simulink model "test_rx_err_cnt"  (Simulink 6.2)
settings: Solver=ode45  StartTime=0.0  StopTime=1000  RelTol=1e-3
libraries: xbsIndex_r3 x58, xps_library x6, casper_library x2
settings Model: LastModifiedBy=dsp
settings DebuggingCC: SolverPrmCheckMsg=warning

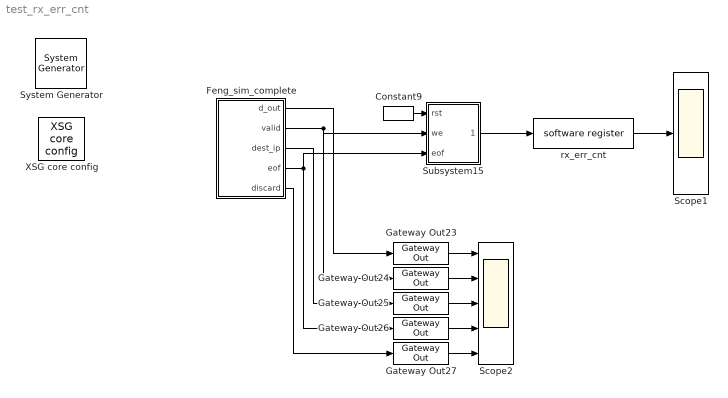
== system test_rx_err_cnt ==
  " System Generator" : xbsIndex_r3/ System Generator  Tag=genX  xilinxfamily=Virtex2P  part=xc2vp70  speed=-7  package=ff1704  synthesis_tool=XST  directory=./b_2x_8a_r308d/sysgen  testbench=off  simulink_period=1  sysclk_period=4.878  incr_netlist=off  trim_vbits=Everywhere in SubSystem  dbl_ovrd=According to Block Masks  core_generation=According to Block Masks  run_coregen=off  deprecated_control=off  eval_field=0
      settings: AttributesFormatString=System\nGenerator
  Constant9 : xbsIndex_r3/Constant  const=0  equ=P=C  arith_type=Boolean  n_bits=1  bin_pt=0  opselect=C  inp2=PCIN>>17  opr=+  inp1=P  carry=CIN  iostate=0  explicit_period=on  period=1  dbl_ovrd=off
  Feng_sim_complete : Subsystem
  Gateway Out{23..27} (5 alike) : xbsIndex_r3/Gateway Out  output_type=Double  nbits=8  bin_pt=6  arith_type=Boolean  quantization=Truncate  overflow=Wrap  hdl_port=on  timing_constraint=None  locs_specified=off  LOCs={}  needs_fixed_name=off  show_param=off
      settings: xl_area=[0, 0, 0, 0, 0, 0, 0]
  Scope1 : Scope
      settings: TimeRange=10000  YMin=0  YMax=5000
  Scope2 : Scope  NumInputPorts=5
      settings: TimeRange=10000  YMin=0~0~0~0~-1  YMax=5000~1~3~1~1
  Subsystem15 : Subsystem  mask{payload_len=51}
      mask init:
      | fmtstr = sprintf('Payload Length: %d', payload_len);
      | set_param(gcb, 'AttributesFormatString', fmtstr);
      settings: AttributesFormatString=Payload Length: 51
  XSG core config : xps_library/XSG core config  Tag=xps:xsg  hw_sys=BEE2_usr  ibob_linux=off  clk_src=sys_clk2x  gpio_clk_io_group=iBOB:sma  gpio_clk_bit_index=0  clk_rate=205  sample_period=1  synthesis_tool=XST  mpc_type=powerpc405
  rx_err_cnt : xps_library/software register  Tag=xps:sw_reg  io_dir=To Processor  arith_type=Unsigned  bitwidth=32  bin_pt=0  sample_period=1  gw_name=test_rx_err_cnt_rx_err_cnt_user_data_in
  wires:
  Subsystem15/1(err_cnt) -> rx_err_cnt/1
  Constant9/1 -> Subsystem15/1(rst)
  Gateway Out23/1 -> Scope2/1
  Gateway Out24/1 -> Scope2/2
  Gateway Out25/1 -> Scope2/3
  Gateway Out26/1 -> Scope2/4
  Gateway Out27/1 -> Scope2/5
  Feng_sim_complete/1(d_out) -> Gateway Out23/1
  Feng_sim_complete/2(valid) -> Gateway Out24/1, Subsystem15/2(we)
  Feng_sim_complete/3(dest_ip) -> Gateway Out25/1
  Feng_sim_complete/4(eof) -> Gateway Out26/1, Subsystem15/3(eof)
  Feng_sim_complete/5(discard) -> Gateway Out27/1
  rx_err_cnt/1 -> Scope1/1

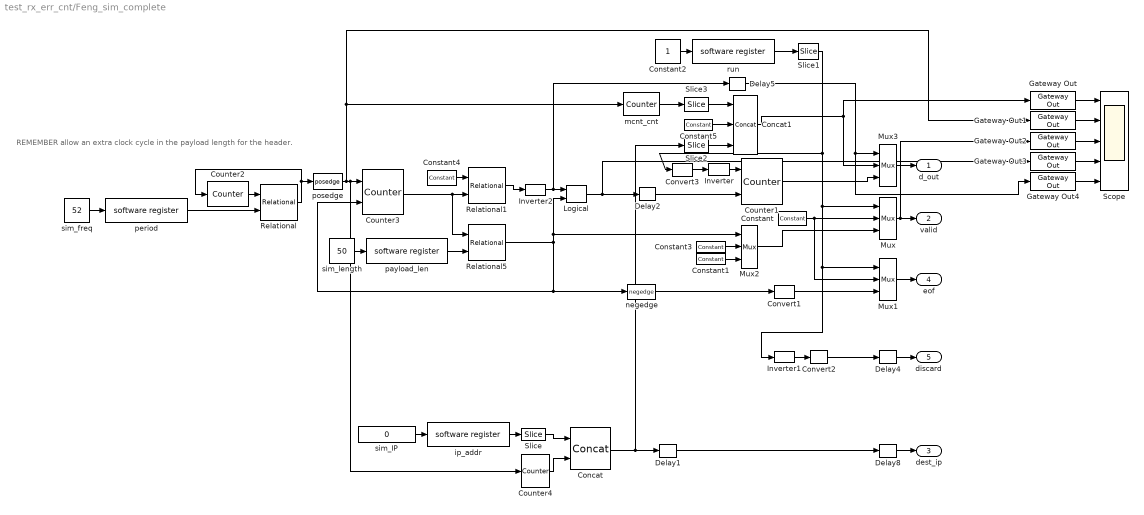
== system test_rx_err_cnt/Feng_sim_complete ==
  note: REMEMBER
      | allow an extra clock cycle in the
      | payload length for the header.
  Concat : xbsIndex_r3/Concat  num_inputs=2  explicit_period=off  period=1  dbl_ovrd=off
  Concat1 : xbsIndex_r3/Concat  num_inputs=3  explicit_period=off  period=1  dbl_ovrd=off
  Constant : xbsIndex_r3/Constant  const=0  equ=P=C  arith_type=Boolean  n_bits=1  bin_pt=0  opselect=C  inp2=PCIN>>17  opr=+  inp1=P  carry=CIN  iostate=0  explicit_period=on  period=1  dbl_ovrd=off
  Constant1 : xbsIndex_r3/Constant  const=1  equ=P=C  arith_type=Boolean  n_bits=1  bin_pt=0  opselect=C  inp2=PCIN>>17  opr=+  inp1=P  carry=CIN  iostate=0  explicit_period=off  period=1  dbl_ovrd=off
  Constant2 : Constant
  Constant3 : xbsIndex_r3/Constant  const=0  equ=P=C  arith_type=Boolean  n_bits=1  bin_pt=0  opselect=C  inp2=PCIN>>17  opr=+  inp1=P  carry=CIN  iostate=0  explicit_period=off  period=1  dbl_ovrd=off
  Constant4 : xbsIndex_r3/Constant  const=0  equ=P=C  arith_type=Unsigned  n_bits=32  bin_pt=0  opselect=C  inp2=PCIN>>17  opr=+  inp1=P  carry=CIN  iostate=0  explicit_period=on  period=1  dbl_ovrd=off
  Constant5 : xbsIndex_r3/Constant  const=0  equ=P=C  arith_type=Unsigned  n_bits=16-2  bin_pt=0  opselect=C  inp2=PCIN>>17  opr=+  inp1=P  carry=CIN  iostate=0  explicit_period=on  period=1  dbl_ovrd=off
  Convert1 : xbsIndex_r3/Convert  arith_type=Boolean  n_bits=8  bin_pt=6  quantization=Truncate  overflow=Wrap  latency=0  explicit_period=on  period=1  dbl_ovrd=off  show_param=off  inserted_by_tool=off  pipeline=off
      settings: xl_area=[0, 0, 0, 0, 0, 0, 0]
  Convert2 : xbsIndex_r3/Convert  arith_type=Boolean  n_bits=8  bin_pt=6  quantization=Truncate  overflow=Wrap  latency=0  explicit_period=on  period=1  dbl_ovrd=off  show_param=off  inserted_by_tool=off  pipeline=off
      settings: xl_area=[0, 0, 0, 0, 0, 0, 0]
  Convert3 : xbsIndex_r3/Convert  arith_type=Boolean  n_bits=8  bin_pt=6  quantization=Truncate  overflow=Wrap  latency=0  explicit_period=on  period=1  dbl_ovrd=off  show_param=off  inserted_by_tool=off  pipeline=off
      settings: xl_area=[0, 0, 0, 0, 0, 0, 0]
  Counter1 : xbsIndex_r3/Counter  cnt_type=Free Running  n_bits=64  bin_pt=0  arith_type=Unsigned  start_count=0  cnt_to=Inf  cnt_by_val=1  operation=Up  explicit_period=off  period=1  load_pin=off  rst=on  en=on  dbl_ovrd=off  show_param=off  use_rpm=off  gen_core=off
      settings: xl_area=[0, 0, 0, 0, 0, 0, 0]
  Counter2 : xbsIndex_r3/Counter  cnt_type=Free Running  n_bits=32  bin_pt=0  arith_type=Unsigned  start_count=1  cnt_to=Inf  cnt_by_val=1  operation=Up  explicit_period=on  period=1  load_pin=off  rst=on  en=off  dbl_ovrd=off  show_param=off  use_rpm=on  gen_core=off
      settings: xl_area=[0, 0, 0, 0, 0, 0, 0]
  Counter3 : xbsIndex_r3/Counter  cnt_type=Free Running  n_bits=32  bin_pt=0  arith_type=Unsigned  start_count=0  cnt_to=1023  cnt_by_val=1  operation=Up  explicit_period=on  period=1  load_pin=off  rst=on  en=on  dbl_ovrd=off  show_param=off  use_rpm=on  gen_core=off
      settings: xl_area=[0, 0, 0, 0, 0, 0, 0]
  Counter4 : xbsIndex_r3/Counter  cnt_type=Free Running  n_bits=2  bin_pt=0  arith_type=Unsigned  start_count=0  cnt_to=1023  cnt_by_val=1  operation=Up  explicit_period=on  period=1  load_pin=off  rst=off  en=on  dbl_ovrd=off  show_param=off  use_rpm=on  gen_core=off
      settings: xl_area=[0, 0, 0, 0, 0, 0, 0]
  Delay{1..2,4..5,8} (5 alike) : xbsIndex_r3/Delay  latency=1  reg_retiming=on  explicit_period=off  period=1  en=off  accept_only_valid=off  init_zero=on  dbl_ovrd=off  show_param=off
      settings: xl_area=[0, 0, 0, 0, 0, 0, 0]
  Gateway Out{,1..4} (5 alike) : xbsIndex_r3/Gateway Out  output_type=Double  nbits=8  bin_pt=6  arith_type=Boolean  quantization=Truncate  overflow=Wrap  hdl_port=on  timing_constraint=None  locs_specified=off  LOCs={}  needs_fixed_name=off  show_param=off
      settings: xl_area=[0, 0, 0, 0, 0, 0, 0]
  Inverter : xbsIndex_r3/Inverter  latency=0  explicit_period=off  period=1  en=off  dbl_ovrd=off  show_param=off
      settings: xl_area=[0, 0, 0, 0, 0, 0, 0]
  Inverter1 : xbsIndex_r3/Inverter  latency=0  explicit_period=off  period=1  en=off  dbl_ovrd=off  show_param=off
      settings: xl_area=[0, 0, 0, 0, 0, 0, 0]
  Inverter2 : xbsIndex_r3/Inverter  latency=0  explicit_period=off  period=1  en=off  dbl_ovrd=off  show_param=off
      settings: xl_area=[0, 0, 0, 0, 0, 0, 0]
  Logical : xbsIndex_r3/Logical  logical_function=AND  inputs=2  precision=Full  arith_type=Unsigned  n_bits=8  bin_pt=2  align_bp=on  latency=0  explicit_period=off  period=1  en=off  dbl_ovrd=off  show_param=off
      settings: xl_area=[0, 0, 0, 0, 0, 0, 0]
  Mux{,1..3} (4 alike) : xbsIndex_r3/Mux  inputs=2  precision=Full  arith_type="Signed  (2's comp)"  n_bits=8  bin_pt=2  quantization=Truncate  overflow=Wrap  latency=1  explicit_period=off  period=1  en=off  dbl_ovrd=off  show_param=off  mux_type=off  use_rpm=off  gen_core=off
      settings: xl_area=[0, 0, 0, 0, 0, 0, 0]
  Relational : xbsIndex_r3/Relational  mode=a>=b  latency=0  explicit_period=on  period=1  en=off  dbl_ovrd=off  show_param=off
      settings: xl_area=[0, 0, 0, 0, 0, 0, 0]
  Relational1 : xbsIndex_r3/Relational  mode=a=b  latency=0  explicit_period=off  period=1  en=off  dbl_ovrd=off  show_param=off
      settings: xl_area=[0, 0, 0, 0, 0, 0, 0]
  Relational5 : xbsIndex_r3/Relational  mode=a<=b  latency=0  explicit_period=off  period=1  en=off  dbl_ovrd=off  show_param=off
      settings: xl_area=[0, 0, 0, 0, 0, 0, 0]
  Scope : Scope  NumInputPorts=5
      settings: TimeRange=4000  YMin=130000~0~0~0~0  YMax=200000~1~1~1~1  SaveName=ScopeData11
  Slice : xbsIndex_r3/Slice  mode=Upper Bit Location + Width  nbits=30  bit1=0  base1=MSB of Input  bit0=0  base0=LSB of Input  boolean_output=off  explicit_period=off  period=1  dbl_ovrd=off
  Slice1 : xbsIndex_r3/Slice  mode=Lower Bit Location + Width  nbits=1  bit1=1  base1=MSB of Input  bit0=0  base0=LSB of Input  boolean_output=off  explicit_period=off  period=1  dbl_ovrd=off
  Slice2 : xbsIndex_r3/Slice  mode=Lower Bit Location + Width  nbits=2  bit1=1  base1=MSB of Input  bit0=0  base0=LSB of Input  boolean_output=off  explicit_period=off  period=1  dbl_ovrd=off
  Slice3 : xbsIndex_r3/Slice  mode=Lower Bit Location + Width  nbits=48  bit1=1  base1=MSB of Input  bit0=3  base0=LSB of Input  boolean_output=off  explicit_period=off  period=1  dbl_ovrd=off
  ip_addr : xps_library/software register  Tag=xps:sw_reg  io_dir=From Processor  arith_type=Unsigned  bitwidth=32  bin_pt=0  sample_period=1  gw_name=test_rx_err_cnt_Feng_sim_complete_ip_addr_user_data_out
  mcnt_cnt : xbsIndex_r3/Counter  cnt_type=Free Running  n_bits=64  bin_pt=0  arith_type=Unsigned  start_count=0  cnt_to=Inf  cnt_by_val=1  operation=Up  explicit_period=off  period=1  load_pin=off  rst=off  en=on  dbl_ovrd=off  show_param=off  use_rpm=off  gen_core=off
      settings: xl_area=[0, 0, 0, 0, 0, 0, 0]
  negedge : casper_library/Misc/negedge  Tag=Rising Edge Detector
  payload_len : xps_library/software register  Tag=xps:sw_reg  io_dir=From Processor  arith_type=Unsigned  bitwidth=32  bin_pt=0  sample_period=1  gw_name=test_rx_err_cnt_Feng_sim_complete_payload_len_user_data_out
  period : xps_library/software register  Tag=xps:sw_reg  io_dir=From Processor  arith_type=Unsigned  bitwidth=32  bin_pt=0  sample_period=1  gw_name=test_rx_err_cnt_Feng_sim_complete_period_user_data_out
  posedge : casper_library/Misc/pulse_ext/posedge  Tag=Rising Edge Detector
  run : xps_library/software register  Tag=xps:sw_reg  io_dir=From Processor  arith_type=Unsigned  bitwidth=32  bin_pt=0  sample_period=1  gw_name=test_rx_err_cnt_Feng_sim_complete_run_user_data_out
  sim_IP : Constant  Value=0
  sim_freq : Constant  Value=52
  sim_length : Constant  Value=50
  d_out : Outport
  valid : Outport  Port=2
  dest_ip : Outport  Port=3
  eof : Outport  Port=4
  discard : Outport  Port=5
  wires:
  Delay1/1 -> Delay8/1
  Slice2/1 -> Concat1/3
  Slice3/1 -> Concat1/1
  Logical/1 -> Gateway Out3/1, Delay2/1
  Gateway Out4/1 -> Scope/5
  Gateway Out3/1 -> Scope/4
  Gateway Out2/1 -> Scope/3
  Gateway Out1/1 -> Scope/2
  Gateway Out/1 -> Scope/1
  Delay5/1 -> Gateway Out4/1, Mux3/1
  Concat1/1 -> Gateway Out/1, Mux3/2
  Constant5/1 -> Concat1/2
  mcnt_cnt/1 -> Slice3/1
  Inverter2/1 -> Logical/1, Delay5/1
  Relational1/1 -> Inverter2/1
  Constant4/1 -> Relational1/1
  Concat/1 -> Slice2/1, Delay1/1
  Slice/1 -> Concat/1
  Counter4/1 -> Concat/2
  ip_addr/1 -> Slice/1
  Convert2/1 -> Delay4/1
  Inverter1/1 -> Convert2/1
  Constant1/1 -> Mux2/3
  Constant3/1 -> Mux2/2
  Convert3/1 -> Inverter/1
  Delay2/1 -> Counter1/2
  Inverter/1 -> Counter1/1
  Mux2/1 -> Mux/3
  Delay4/1 -> discard/1
  Slice1/1 -> Convert3/1, Inverter1/1, Mux1/1, Mux/1
  Constant2/1 -> run/1
  run/1 -> Slice1/1
  Delay8/1 -> dest_ip/1
  Mux3/1 -> d_out/1
  Convert1/1 -> Mux1/3
  Mux1/1 -> eof/1
  Constant/1 -> Mux1/2, Mux/2
  Mux/1 -> Gateway Out2/1, valid/1
  payload_len/1 -> Relational5/2
  sim_length/1 -> payload_len/1
  posedge/1 -> Gateway Out1/1, mcnt_cnt/1, Counter4/1, Counter3/1
  Counter3/1 -> Relational1/2, Relational5/1
  Relational5/1 -> Counter3/2, negedge/1, Mux2/1, Logical/2
  sim_IP/1 -> ip_addr/1
  sim_freq/1 -> period/1
  period/1 -> Relational/2
  negedge/1 -> Convert1/1
  Counter1/1 -> Mux3/3
  Relational/1 -> Counter2/1, posedge/1
  Counter2/1 -> Relational/1

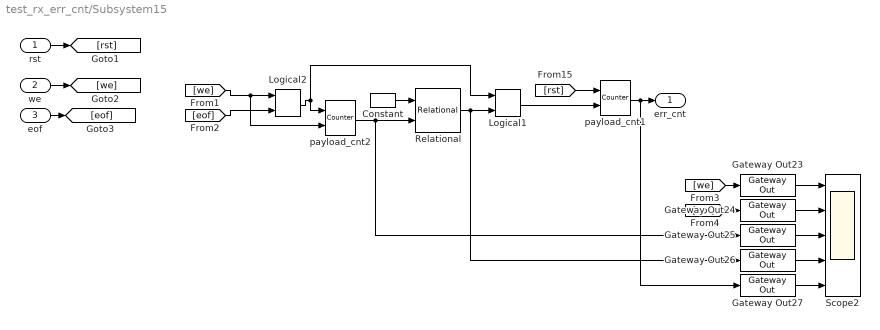
== system test_rx_err_cnt/Subsystem15 ==
  rst : Inport  Port=1  LatchInput=off
  we : Inport  Port=2  LatchInput=off
  eof : Inport  Port=3  LatchInput=off
  Constant : xbsIndex_r3/Constant  const=payload_len -1  equ=P=C  arith_type=Unsigned  n_bits=8  bin_pt=0  opselect=C  inp2=PCIN>>17  opr=+  inp1=P  carry=CIN  iostate=0  explicit_period=off  period=1  dbl_ovrd=off
  Gateway Out{23..27} (5 alike) : xbsIndex_r3/Gateway Out  output_type=Double  nbits=8  bin_pt=6  arith_type=Boolean  quantization=Truncate  overflow=Wrap  hdl_port=on  timing_constraint=None  locs_specified=off  LOCs={}  needs_fixed_name=off  show_param=off
      settings: xl_area=[0, 0, 0, 0, 0, 0, 0]
  Logical1 : xbsIndex_r3/Logical  logical_function=AND  inputs=2  precision=Full  arith_type=Unsigned  n_bits=8  bin_pt=2  align_bp=on  latency=0  explicit_period=on  period=1  en=off  dbl_ovrd=off  show_param=off
      settings: xl_area=[0, 0, 0, 0, 0, 0, 0]
  Logical2 : xbsIndex_r3/Logical  logical_function=AND  inputs=2  precision=Full  arith_type=Unsigned  n_bits=8  bin_pt=2  align_bp=on  latency=0  explicit_period=on  period=1  en=off  dbl_ovrd=off  show_param=off
      settings: xl_area=[0, 0, 0, 0, 0, 0, 0]
  Relational : xbsIndex_r3/Relational  mode=a!=b  latency=0  explicit_period=off  period=1  en=off  dbl_ovrd=off  show_param=off
      settings: xl_area=[0, 0, 0, 0, 0, 0, 0]
  Scope2 : Scope  NumInputPorts=5
      settings: TimeRange=10000  YMin=0~0~0~0~-1  YMax=5000~1~3~1~1  SaveName=ScopeData2
  payload_cnt1 : xbsIndex_r3/Counter  cnt_type=Free Running  n_bits=32  bin_pt=0  arith_type=Unsigned  start_count=0  cnt_to=0  cnt_by_val=1  operation=Up  explicit_period=on  period=1  load_pin=off  rst=on  en=on  dbl_ovrd=off  show_param=off  use_rpm=on  gen_core=off
      settings: xl_area=[0, 0, 0, 0, 0, 0, 0]
  payload_cnt2 : xbsIndex_r3/Counter  cnt_type=Free Running  n_bits=8  bin_pt=0  arith_type=Unsigned  start_count=0  cnt_to=0  cnt_by_val=1  operation=Up  explicit_period=on  period=1  load_pin=off  rst=on  en=on  dbl_ovrd=off  show_param=off  use_rpm=on  gen_core=off
      settings: xl_area=[0, 0, 0, 0, 0, 0, 0]
  err_cnt : Outport
  wires:
  payload_cnt1/1 -> err_cnt/1, Gateway Out27/1
  rst/1 -> [rst]
  [rst] -> payload_cnt1/1
  we/1 -> [we]
  eof/1 -> [eof]
  Logical2/1 -> payload_cnt2/1, Logical1/1
  payload_cnt2/1 -> Relational/2, Gateway Out25/1
  [we] -> Logical2/1, payload_cnt2/2
  [eof] -> Logical2/2
  Constant/1 -> Relational/1
  Relational/1 -> Logical1/2, Gateway Out26/1
  Logical1/1 -> payload_cnt1/2
  Gateway Out23/1 -> Scope2/1
  Gateway Out24/1 -> Scope2/2
  Gateway Out25/1 -> Scope2/3
  Gateway Out26/1 -> Scope2/4
  Gateway Out27/1 -> Scope2/5
  [we] -> Gateway Out23/1
  [eof] -> Gateway Out24/1
